simulink model "ejector"  (R2024b)
settings: Solver=VariableStepAuto  StartTime=0.0  StopTime=60  RelTol=1e-3
settings Model: Creator=10537  LastModifiedBy=10537

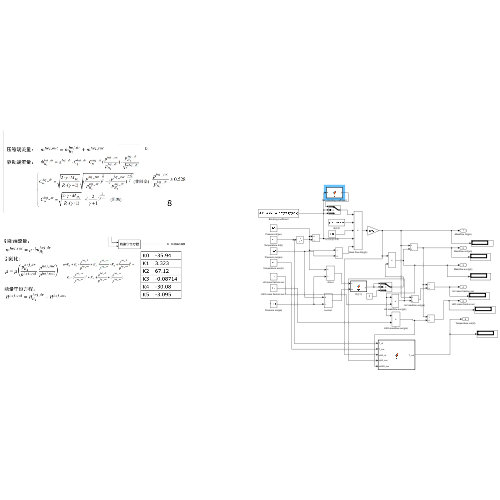
[thumbnail: Simulink's stored preview of the top-level diagram]
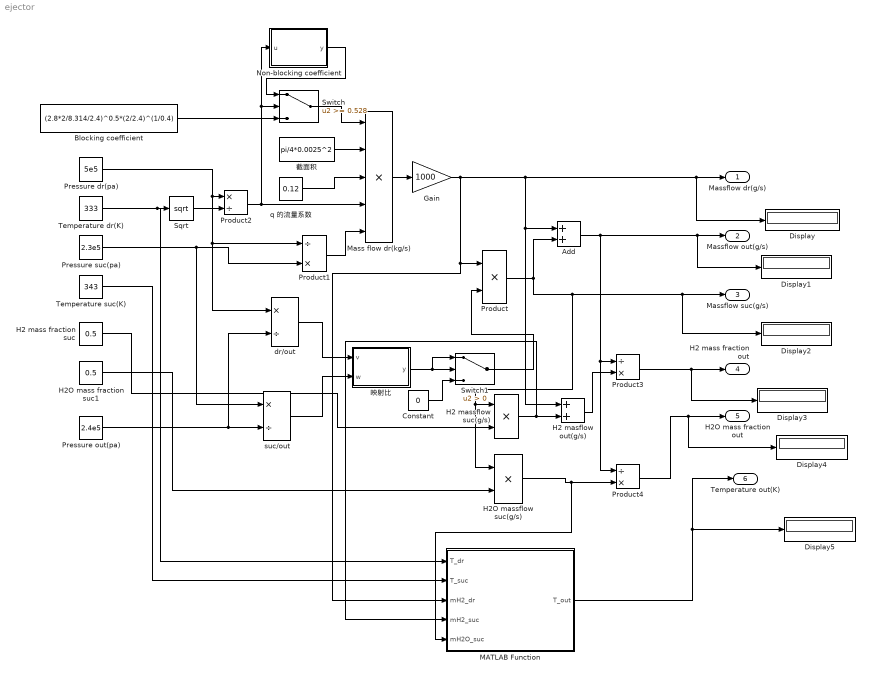
== system ejector ==
  Add : Sum
  Blocking coefficient : Constant  Value=(2.8*2/8.314/2.4)^0.5*(2/2.4)^(1/0.4)
  Constant : Constant  Value=0
  Display{,1..5} (6 alike) : Display
  Gain : Gain  Gain=1000
  H2 masflow out(g/s) : Sum
  H2 mass fraction suc : Constant  Value=0.5
  H2 massflow suc(g/s) : Product
  H2O mass fraction suc1 : Constant  Value=0.5
  H2O massflow suc(g/s) : Product  Inputs=**
  MATLAB Function : MATLAB Function  TreatAsAtomicUnit=on
  Mass flow dr(kg/s) : Product  Inputs=5
  Non-blocking coefficient : MATLAB Function  TreatAsAtomicUnit=on
  Pressure dr(pa) : Constant  Value=5e5
  Pressure out(pa) : Constant  Value=2.4e5
  Pressure suc(pa) : Constant  Value=2.3e5
  Product : Product
  Product1 : Product  Inputs=/*
  Product2 : Product  Inputs=*/
  Product3 : Product  Inputs=/*
  Product4 : Product  Inputs=/*
  Sqrt : Sqrt
  Switch : Switch  Threshold=0.528  SaturateOnIntegerOverflow=off  InputSameDT=off
  Switch1 : Switch  Criteria=u2 > Threshold  SaturateOnIntegerOverflow=off  InputSameDT=off
  Temperature dr(K) : Constant  Value=333
  Temperature suc(K) : Constant  Value=343
  dr/out : Product  Inputs=*/
  q 的流量系数 : Constant  Value=0.12
  suc/out : Product  Inputs=*/
  截面积 : Constant  Value=pi/4*0.0025^2
  映射比 : MATLAB Function  TreatAsAtomicUnit=on
  Massflow dr(g/s) : Outport
  Massflow out(g/s) : Outport  Port=2
  Massflow suc(g/s) : Outport  Port=3
  H2 mass fraction out : Outport  Port=4
  H2O mass fraction out : Outport  Port=5
  Temperature out(K) : Outport  Port=6
  wires:
  Pressure dr(pa)/1 -> dr/out/1, Product1/1, Product2/1
  Pressure suc(pa)/1 -> suc/out/1, Product1/2
  Temperature dr(K)/1 -> Sqrt/1, MATLAB Function/1(T_dr)
  Product1/1 -> Mass flow dr(kg/s)/5
  Sqrt/1 -> Product2/2
  Product2/1 -> Non-blocking coefficient/1(u), Switch/2, Mass flow dr(kg/s)/4
  q 的流量系数/1 -> Mass flow dr(kg/s)/3
  截面积/1 -> Mass flow dr(kg/s)/2
  Switch/1 -> Mass flow dr(kg/s)/1
  Blocking coefficient/1 -> Switch/3
  Non-blocking coefficient/1(y) -> Switch/1
  Mass flow dr(kg/s)/1 -> Gain/1
  Gain/1 -> H2 masflow out(g/s)/1, Add/1, Display/1, Massflow dr(g/s)/1, MATLAB Function/3(mH2_dr), Product/1
  Pressure out(pa)/1 -> dr/out/2, suc/out/2
  dr/out/1 -> 映射比/1(v)
  suc/out/1 -> 映射比/2(w)
  映射比/1(y) -> Switch1/1, Switch1/2
  Constant/1 -> Switch1/3
  Switch1/1 -> Product/2
  Product/1 -> Add/2, H2O massflow suc(g/s)/1, H2 massflow suc(g/s)/1, Display2/1, Massflow suc(g/s)/1
  Add/1 -> Display1/1, Massflow out(g/s)/1, Product4/1, Product3/1
  H2 mass fraction suc/1 -> H2 massflow suc(g/s)/2
  H2O mass fraction suc1/1 -> H2O massflow suc(g/s)/2
  H2 massflow suc(g/s)/1 -> MATLAB Function/4(mH2_suc), H2 masflow out(g/s)/2
  H2 masflow out(g/s)/1 -> Product3/2
  H2O massflow suc(g/s)/1 -> MATLAB Function/5(mH2O_suc), Product4/2
  Product4/1 -> Display4/1, H2O mass fraction out/1
  Temperature suc(K)/1 -> MATLAB Function/2(T_suc)
  MATLAB Function/1(T_out) -> Display5/1, Temperature out(K)/1
  Product3/1 -> Display3/1, H2 mass fraction out/1

== matlab function ejector/映射比 ==
  data: v input; y output; w input
function y = fcn(v,w)
%#codegen

y = -35.94+3.323*v+67.12*w-0.08714*v*v-30.08*w*w-3.095*v*w;

== matlab function ejector/Non-blocking coefficient ==
  data: u input; y output
function y = fcn(u)
a = (2*1.4*2/8.314/0.4)^0.5;
b = sqrt(abs(u^(2/1.4) - u^(2.4/1.4)));
%b = (u^(2/1.4)-u^(2.4/1.4))^0.5;
y = a*b;

== matlab function ejector/MATLAB Function ==
  data: T_dr input; T_out output; T_suc input; mH2_dr input; mH2_suc input; mH2O_suc input
function T_out = fcn(T_dr,T_suc,mH2_dr,mH2_suc,mH2O_suc)
H_dr=14.3*mH2_dr*T_dr;
H_suc=14.3*mH2_suc*T_suc+1.85*mH2O_suc*T_suc;
mH2_out=mH2_suc+mH2_dr;
T_out=(H_dr+H_suc)/(14.3*mH2_out+1.85*mH2O_suc+0.0000001);
